simulink model "example_no_divide_by_zeroFcn"  (Simulink 7.4)
settings: Solver=ode45  StartTime=0.0  StopTime=10.0  RelTol=1e-3
settings Model: Creator=rabdul  LastModifiedBy=ssasikum
settings DebuggingCC: StrictBusMsg=ErrorLevel1

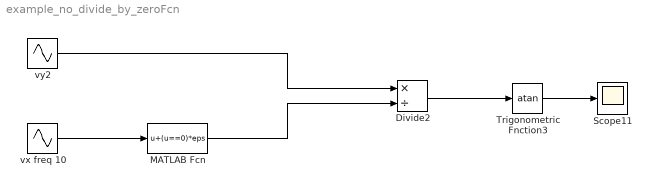
== system example_no_divide_by_zeroFcn ==
  Divide2 : Product  Inputs=*/
  MATLAB Fcn : MATLABFcn  MATLABFcn=u+(u==0)*eps
  Scope11 : Scope
  Trigonometric Fnction3 : Trigonometry  Operator=atan
  vx freq 10 : Sin  Amplitude=1  Bias=0  Frequency=10  Phase=0  Samples=10  SampleTime=0  Offset=0
  vy2 : Sin  Amplitude=1  Bias=0  Frequency=10  Phase=0.2  Samples=10  SampleTime=0  Offset=0
  wires:
  vy2/1 -> Divide2/1
  Divide2/1 -> Trigonometric Fnction3/1
  Trigonometric Fnction3/1 -> Scope11/1
  vx freq 10/1 -> MATLAB Fcn/1
  MATLAB Fcn/1 -> Divide2/2
